simulink model "HDVSim_Dual_Fuel_Hybrid_Truck"  (R2018b)
settings: Solver=ode3  StartTime=0.0  StopTime=inf  FixedStep=sample_time  MaxStep=0.1  RelTol=1e-3  EnableMultiTasking=on
model workspace (MAT data in the model file):
  Bat : struct (value not decoded)
  Electric_Truck = 0
  Fueltype = 11
  Hybrid_Truck = 1
  IZ12 = 3600
  SOC_T_EM_completely_available = 0.089152566
  SOC_addition = 0.262901104
  SOC_target = 0
  Sailing_without_drag_torque = 1
  MCOS : class17 (value not decoded)
  TCO_Trailer = 1
  T_distance_LPS_down = 500
  T_distance_LPS_up = 434.9496342
  VSim : struct (value not decoded)
  Vehicle = 'LNGDieselHybrid'
  WPT : struct (value not decoded)
  MCOS : class17 (value not decoded)
  addition_for_critical_slope = 0.030662181
  ambient : struct (value not decoded)
  auxiliary_consumers : struct (value not decoded)
  critical_altitude_difference = 39.0505026
  cycle : struct (value not decoded)
  dcycle = 5
  distance_1_PPC = 130
  distance_2_PPC = 290
  distance_PPC_altitude_difference = 4273.353363
  driver : struct (value not decoded)
  em : struct (value not decoded)
  engine : struct (value not decoded)
  final_drive : struct (value not decoded)
  ifElectric = 0
  ifOptimized = 1
  look_ahead_PPC = 920
  max_distance = 3000
  name = 'HDVSim_Dual_Fuel_Hybrid_Truck'
  preditiveCruiseControl = 1
  sample_time = 0.1
  tank : struct (value not decoded)
  tires : struct (value not decoded)
  transmission : struct (value not decoded)
  v_PPC_delta = 2.77123754361
  v_max_electrical_drive_only = 9.22694367778
  vehicle : struct (value not decoded)
  MCOS : class17 (value not decoded)
  MCOS : class17 (value not decoded)
  x = [17.07936487 6 0 0 2.860669464 1810.391452 1020.247354 1265.144022 9.976455157 83 4 20 ... (27 elements, 1x27)]
values from neighbouring files (symbols this model uses):
  transmission = Transmission_gearing(1, 1, false, false, final_drive.ratio)    [Parameterizing.m]
symbols that are objects in the model workspace (value not decoded): ambient, auxiliary_consumers, Bat, cycle, driver, em, engine, final_drive, tires, vehicle
undefined symbols (not defined in the file or in its folder): Hybrid_LKW, Ion, Lithium
libraries: simulink x22, powerlib x2, electricdrivelib x1
(part 2 of 3)

== system HDVSim_Dual_Fuel_Hybrid_Truck/Active cruise control/Estimate acceleration ==
  v_target [m/s] : Inport
  Slope_0 : Inport  Port=2
  Slope_50 : Inport  Port=3
  Slope_100 : Inport  Port=4
  Slope_150 : Inport  Port=5
  Slope_200 : Inport  Port=6
  "Steigung_250 " : Inport  Port=7
  Slope_300 : Inport  Port=8
  Slope_350 : Inport  Port=9
  Slope_400 : Inport  Port=10
  Slope_450 : Inport  Port=11
  Add4 : Sum
  Constant4 : Constant  Value=vehicle.payload
  Constant9 : Constant  Value=vehicle.mass
  Demux : Demux  Outputs=10
  Divide1 : Product  Inputs=*/
  Driving resistance without acceleration : Subsystem
  Gain1 : Gain  Gain=-1
  Mux : Mux  Inputs=10
  Trigonometric Function2 : Trigonometry  Operator=atan
  Acceleration_0 : Outport
  Acceleration_50 : Outport  Port=2
  Acceleration_100 : Outport  Port=3
  Acceleration_150 : Outport  Port=4
  Acceleration_200 : Outport  Port=5
  Acceleration_250 : Outport  Port=6
  Acceleration_300 : Outport  Port=7
  Acceleration_350 : Outport  Port=8
  Acceleration_400 : Outport  Port=9
  Acceleration_450 : Outport  Port=10
  wires:
  v_target [m/s]/1 -> Driving resistance without acceleration/1(v [m/s])
  Trigonometric Function2/1 -> Driving resistance without acceleration/2(alpha [rad])
  Constant9/1 -> Add4/1
  Constant4/1 -> Add4/2
  Driving resistance without acceleration/1(F_x (resist) [N]) -> Gain1/1
  Add4/1 -> Divide1/2
  Gain1/1 -> Divide1/1
  Mux/1 -> Trigonometric Function2/1
  Divide1/1 -> Demux/1
  Demux/1 -> Acceleration_0/1
  Slope_0/1 -> Mux/1
  Slope_50/1 -> Mux/2
  Slope_100/1 -> Mux/3
  Slope_150/1 -> Mux/4
  Slope_200/1 -> Mux/5
  "Steigung_250 "/1 -> Mux/6
  Slope_300/1 -> Mux/7
  Slope_350/1 -> Mux/8
  Slope_400/1 -> Mux/9
  Slope_450/1 -> Mux/10
  Demux/2 -> Acceleration_50/1
  Demux/3 -> Acceleration_100/1
  Demux/4 -> Acceleration_150/1
  Demux/5 -> Acceleration_200/1
  Demux/6 -> Acceleration_250/1
  Demux/7 -> Acceleration_300/1
  Demux/8 -> Acceleration_350/1
  Demux/9 -> Acceleration_400/1
  Demux/10 -> Acceleration_450/1

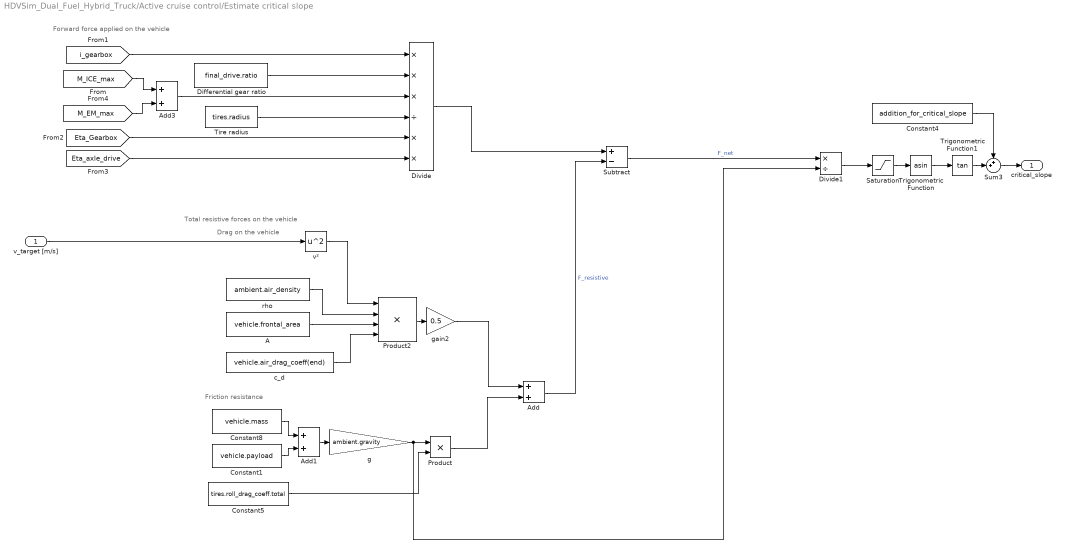
== system HDVSim_Dual_Fuel_Hybrid_Truck/Active cruise control/Estimate critical slope ==
  note: Total resistive forces on the vehicle
  note: Friction resistance
  note: Drag on the vehicle
  note: Forward force applied on the vehicle
  v_target [m/s] : Inport
  A : Constant  Value=vehicle.frontal_area
  Add : Sum
  Add1 : Sum
  Add3 : Sum
  Constant1 : Constant  Value=vehicle.payload
  Constant4 : Constant  Value=addition_for_critical_slope
  Constant5 : Constant  Value=tires.roll_drag_coeff.total
  Constant8 : Constant  Value=vehicle.mass
  Differential gear ratio : Constant  Value=final_drive.ratio
  Divide : Product  Inputs=***/**
  Divide1 : Product  Inputs=*/
  Product : Product
  Product2 : Product  Inputs=4  RndMeth=Zero
  Saturation : Saturate  UpperLimit=1  LowerLimit=-1
  Subtract : Sum  Inputs=+-
  Sum3 : Sum  Inputs=++|
  Tire radius : Constant  Value=tires.radius
  Trigonometric Function : Trigonometry  Operator=asin
  Trigonometric Function1 : Trigonometry  Operator=tan
  c_d : Constant  Value=vehicle.air_drag_coeff(end)
  g : Gain  Gain=ambient.gravity
  gain2 : Gain  Gain=0.5
  rho : Constant  Value=ambient.air_density
  v² : Math  Operator=square  SaturateOnIntegerOverflow=on
  critical_slope : Outport
  wires:
  Add3/1 -> Divide/3
  [i_gearbox] -> Divide/1
  Differential gear ratio/1 -> Divide/2
  Tire radius/1 -> Divide/4
  Divide/1 -> Subtract/1
  Subtract/1 -> Divide1/1  "F_net"
  v²/1 -> Product2/1
  rho/1 -> Product2/2
  A/1 -> Product2/3
  c_d/1 -> Product2/4
  Product2/1 -> gain2/1
  Constant8/1 -> Add1/1
  Constant1/1 -> Add1/2
  Add1/1 -> g/1
  Constant5/1 -> Product/2
  Trigonometric Function/1 -> Trigonometric Function1/1
  Divide1/1 -> Saturation/1
  Sum3/1 -> critical_slope/1
  Constant4/1 -> Sum3/1
  Trigonometric Function1/1 -> Sum3/2
  v_target [m/s]/1 -> v²/1
  [Eta_Gearbox] -> Divide/5
  [Eta_axle_drive] -> Divide/6
  [M_ICE_max] -> Add3/1
  [M_EM_max] -> Add3/2
  gain2/1 -> Add/1
  Product/1 -> Add/2
  Add/1 -> Subtract/2  "F_resistive"
  g/1 -> Product/1, Divide1/2
  Saturation/1 -> Trigonometric Function/1

== system HDVSim_Dual_Fuel_Hybrid_Truck/Active cruise control_old/Braking from upper speed limit ==
  v_soll [m/s] : Inport
  Add3 : Sum  Inputs=+-
  Constant1 : Constant  Value=90/3.6
  Constant10 : Constant  Value=preditiveCruiseControl
  Constant6 : Constant  Value=v_PPC_delta
  Constant7 : Constant  Value=0
  Constant8 : Constant  Value=0
  Saturation Dynamic : simulink/Discontinuities/Saturation Dynamic  OutMin=[]  OutMax=[]  OutDataTypeStr=Inherit: Same as second input  OutDataType=fixdt(1, 16)  OutScaling=2^-10  DoSatur=off
  Switch3 : Switch  Criteria=u2 > Threshold
  Out1 : Outport
  wires:
  Switch3/1 -> Out1/1
  Constant6/1 -> Saturation Dynamic/2
  Constant1/1 -> Add3/1
  Constant7/1 -> Switch3/3
  Add3/1 -> Saturation Dynamic/1
  Constant8/1 -> Saturation Dynamic/3
  Constant10/1 -> Switch3/2
  v_soll [m/s]/1 -> Add3/2
  Saturation Dynamic/1 -> Switch3/1

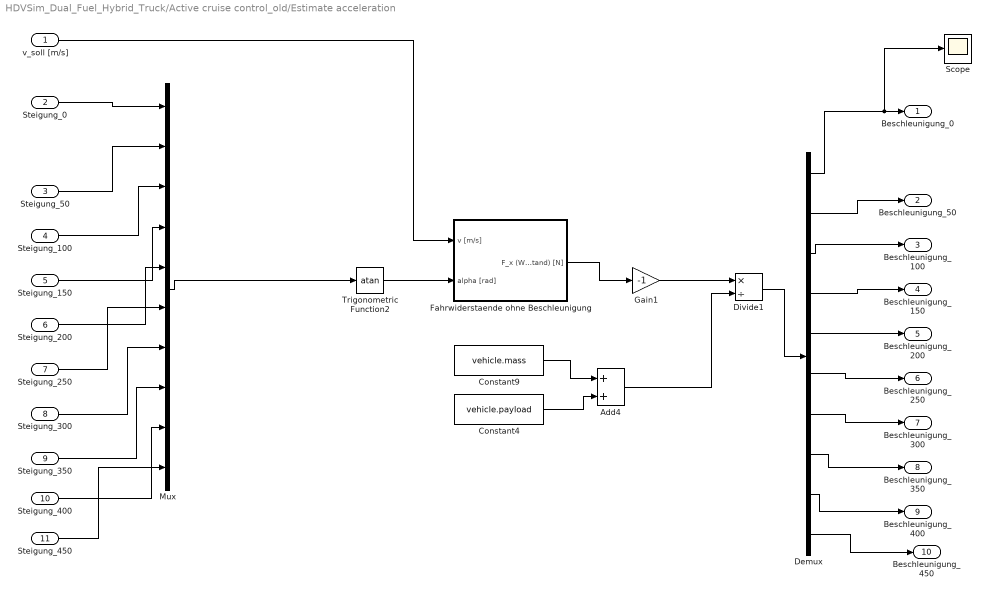
== system HDVSim_Dual_Fuel_Hybrid_Truck/Active cruise control_old/Estimate acceleration ==
  v_soll [m/s] : Inport
  Steigung_0 : Inport  Port=2
  Steigung_50 : Inport  Port=3
  Steigung_100 : Inport  Port=4
  Steigung_150 : Inport  Port=5
  Steigung_200 : Inport  Port=6
  "Steigung_250 " : Inport  Port=7
  Steigung_300 : Inport  Port=8
  Steigung_350 : Inport  Port=9
  Steigung_400 : Inport  Port=10
  Steigung_450 : Inport  Port=11
  Add4 : Sum
  Constant4 : Constant  Value=vehicle.payload
  Constant9 : Constant  Value=vehicle.mass
  Demux : Demux  Outputs=10
  Divide1 : Product  Inputs=*/
  Fahrwiderstaende ohne Beschleunigung : Subsystem
  Gain1 : Gain  Gain=-1
  Mux : Mux  Inputs=10
  Scope : Scope
  Trigonometric Function2 : Trigonometry  Operator=atan
  Beschleunigung_0 : Outport
  Beschleunigung_50 : Outport  Port=2
  Beschleunigung_100 : Outport  Port=3
  Beschleunigung_150 : Outport  Port=4
  Beschleunigung_200 : Outport  Port=5
  Beschleunigung_250 : Outport  Port=6
  Beschleunigung_300 : Outport  Port=7
  Beschleunigung_350 : Outport  Port=8
  Beschleunigung_400 : Outport  Port=9
  Beschleunigung_450 : Outport  Port=10
  wires:
  v_soll [m/s]/1 -> Fahrwiderstaende ohne Beschleunigung/1(v [m/s])
  Trigonometric Function2/1 -> Fahrwiderstaende ohne Beschleunigung/2(alpha [rad])
  Constant9/1 -> Add4/1
  Constant4/1 -> Add4/2
  Fahrwiderstaende ohne Beschleunigung/1(F_x (Widerstand) [N]) -> Gain1/1
  Add4/1 -> Divide1/2
  Gain1/1 -> Divide1/1
  Mux/1 -> Trigonometric Function2/1
  Divide1/1 -> Demux/1
  Demux/1 -> Scope/1, Beschleunigung_0/1
  Steigung_0/1 -> Mux/1
  Steigung_50/1 -> Mux/2
  Steigung_100/1 -> Mux/3
  Steigung_150/1 -> Mux/4
  Steigung_200/1 -> Mux/5
  "Steigung_250 "/1 -> Mux/6
  Steigung_300/1 -> Mux/7
  Steigung_350/1 -> Mux/8
  Steigung_400/1 -> Mux/9
  Steigung_450/1 -> Mux/10
  Demux/2 -> Beschleunigung_50/1
  Demux/3 -> Beschleunigung_100/1
  Demux/4 -> Beschleunigung_150/1
  Demux/5 -> Beschleunigung_200/1
  Demux/6 -> Beschleunigung_250/1
  Demux/7 -> Beschleunigung_300/1
  Demux/8 -> Beschleunigung_350/1
  Demux/9 -> Beschleunigung_400/1
  Demux/10 -> Beschleunigung_450/1

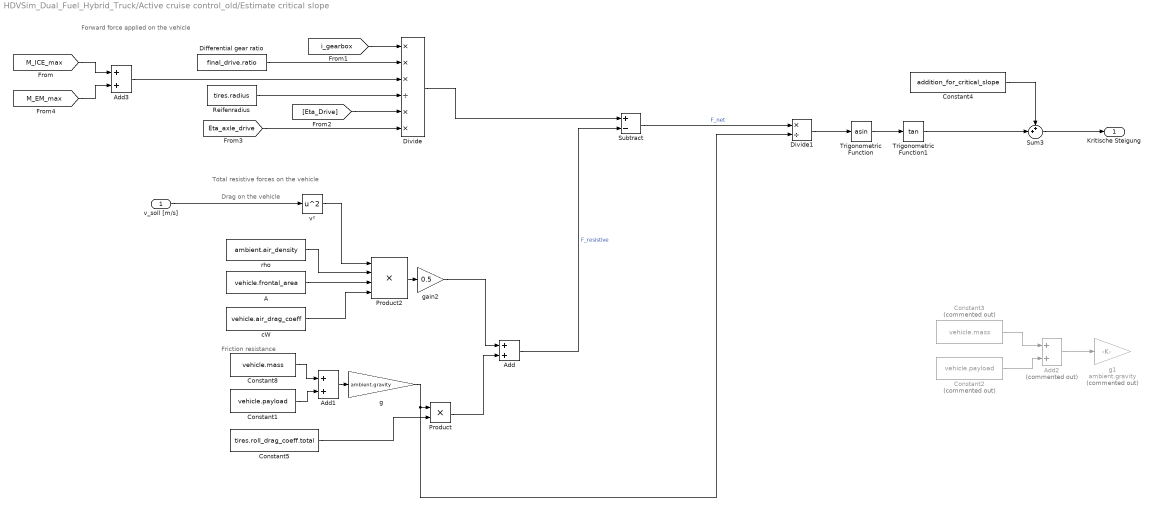
== system HDVSim_Dual_Fuel_Hybrid_Truck/Active cruise control_old/Estimate critical slope ==
  note: Forward force applied on the vehicle
  note: Drag on the vehicle
  note: Friction resistance
  note: Total resistive forces on the vehicle
  v_soll [m/s] : Inport
  A : Constant  Value=vehicle.frontal_area
  Add : Sum
  Add1 : Sum
  Add2 : Sum  Commented=on
  Add3 : Sum
  Constant1 : Constant  Value=vehicle.payload
  Constant2 : Constant  Commented=on  Value=vehicle.payload
  Constant3 : Constant  Commented=on  Value=vehicle.mass
  Constant4 : Constant  Value=addition_for_critical_slope
  Constant5 : Constant  Value=tires.roll_drag_coeff.total
  Constant8 : Constant  Value=vehicle.mass
  Differential gear ratio : Constant  Value=final_drive.ratio
  Divide : Product  Inputs=***/**
  Divide1 : Product  Inputs=*/
  Product : Product
  Product2 : Product  Inputs=4  RndMeth=Zero
  Reifenradius : Constant  Value=tires.radius
  Subtract : Sum  Inputs=+-
  Sum3 : Sum  Inputs=++|
  Trigonometric Function : Trigonometry  Operator=asin
  Trigonometric Function1 : Trigonometry  Operator=tan
  cW : Constant  Value=vehicle.air_drag_coeff
  g : Gain  Gain=ambient.gravity
  g1 : Gain  Commented=on  Gain=ambient.gravity
  gain2 : Gain  Gain=0.5
  rho : Constant  Value=ambient.air_density
  v² : Math  Operator=square  SaturateOnIntegerOverflow=on
  Kritische Steigung : Outport
  wires:
  Add3/1 -> Divide/3
  [i_gearbox] -> Divide/1
  Differential gear ratio/1 -> Divide/2
  Reifenradius/1 -> Divide/4
  Divide/1 -> Subtract/1
  v²/1 -> Product2/1
  rho/1 -> Product2/2
  A/1 -> Product2/3
  cW/1 -> Product2/4
  Product2/1 -> gain2/1
  Constant8/1 -> Add1/1
  Constant1/1 -> Add1/2
  Add1/1 -> g/1
  g/1 -> Divide1/2, Product/1
  Constant5/1 -> Product/2
  Constant3/1 -> Add2/1
  Constant2/1 -> Add2/2
  Add2/1 -> g1/1
  Trigonometric Function/1 -> Trigonometric Function1/1
  Divide1/1 -> Trigonometric Function/1
  Sum3/1 -> Kritische Steigung/1
  Constant4/1 -> Sum3/1
  Trigonometric Function1/1 -> Sum3/2
  v_soll [m/s]/1 -> v²/1
  [Eta_Drive] -> Divide/5
  [Eta_axle_drive] -> Divide/6
  [M_ICE_max] -> Add3/1
  [M_EM_max] -> Add3/2
  gain2/1 -> Add/1
  Product/1 -> Add/2
  Add/1 -> Subtract/2  "F_resistive"
  Subtract/1 -> Divide1/1  "F_net"

== system HDVSim_Dual_Fuel_Hybrid_Truck/Driver controls/PI controller brake ==
  delta_v : Inport
  Add : Sum
  "I - controller " : Gain  Gain=driver.controller_integral_gain
  "Integrator, reset for sign change of delta v" : Integrator  ExternalReset=either  ZeroCross=off
  "P - controller " : Gain  Gain=driver.controller_proportional_gain
  F_target [N] : Outport
  wires:
  "Integrator, reset for sign change of delta v"/1 -> Add/2  "I_part"
  "I - controller "/1 -> "Integrator, reset for sign change of delta v"/1
  Add/1 -> F_target [N]/1  "F_target"
  "P - controller "/1 -> Add/1  "P_part"
  delta_v/1 -> "I - controller "/1, "Integrator, reset for sign change of delta v"/2, "P - controller "/1

== system HDVSim_Dual_Fuel_Hybrid_Truck/Driver controls/PI controller throttle1 ==
  delta_v : Inport
  Add : Sum
  "I - controller " : Gain  Gain=driver.controller_integral_gain
  "Integrator, reset for sign change of delta v" : Integrator  ExternalReset=either  ZeroCross=off
  "P - controller " : Gain  Gain=driver.controller_proportional_gain
  F_target [N] : Outport
  wires:
  "Integrator, reset for sign change of delta v"/1 -> Add/2  "I_part"
  "I - controller "/1 -> "Integrator, reset for sign change of delta v"/1
  Add/1 -> F_target [N]/1  "F_target"
  "P - controller "/1 -> Add/1  "P_partl"
  delta_v/1 -> "Integrator, reset for sign change of delta v"/2, "I - controller "/1, "P - controller "/1

== system HDVSim_Dual_Fuel_Hybrid_Truck/Driver controls/ZKU ==
  In1 : Inport
  Switch1 : Switch  Threshold=1
  zero1 : Constant  Value=0
  Out1 : Outport
  wires:
  zero1/1 -> Switch1/1
  [ZKU] -> Switch1/2
  Switch1/1 -> Out1/1
  In1/1 -> Switch1/3

== system HDVSim_Dual_Fuel_Hybrid_Truck/Driver controls/ZKU1 ==
  In1 : Inport
  Switch1 : Switch  Threshold=1
  zero1 : Constant  Value=0
  Out1 : Outport
  wires:
  In1/1 -> Switch1/3
  Switch1/1 -> Out1/1
  [ZKU] -> Switch1/2
  zero1/1 -> Switch1/1

== system HDVSim_Dual_Fuel_Hybrid_Truck/Driving cycle/Holding time at the beginning ==
  In1 : Inport
  Clock2 : Clock
  Constant3 : Constant  Value=cycle.stop_start
  Constant4 : Constant  Value=0
  Subtract1 : Sum  Inputs=+-
  Switch1 : Switch
  Out1 : Outport
  wires:
  In1/1 -> Switch1/1
  Constant3/1 -> Subtract1/2
  Clock2/1 -> Subtract1/1
  Constant4/1 -> Switch1/3
  Subtract1/1 -> Switch1/2
  Switch1/1 -> Out1/1

== system HDVSim_Dual_Fuel_Hybrid_Truck/Driving cycle/Holding time at the end ==
  In1 : Inport
  Clock1 : Clock
  Constant : Constant
  Constant1 : Constant  Value=cycle.stop_end
  Constant2 : Constant
  Hit Crossing : HitCross  HitCrossingDirection=rising
  Integrator : Integrator  ExternalReset=rising
  Subtract : Sum  Inputs=+-
  Sum1 : Sum  Inputs=|++
  Switch : Switch  Criteria=u2 > Threshold  Threshold=cycle.stop_end
  Out1 : Outport
  wires:
  In1/1 -> Integrator/2
  Constant/1 -> Integrator/1
  Subtract/1 -> Hit Crossing/1
  Integrator/1 -> Switch/1
  Hit Crossing/1 -> Out1/1
  Clock1/1 -> Switch/2
  Constant1/1 -> Sum1/2, Subtract/2
  Sum1/1 -> Switch/3
  Switch/1 -> Subtract/1
  Constant2/1 -> Sum1/1

== system HDVSim_Dual_Fuel_Hybrid_Truck/Driving cycle/Significant speed deviation ==
  In1 : Inport
  Clock : Clock
  Compare To Constant : simulink/Logic and Bit Operations/Compare To Constant  relop=>=  const=30  OutDataTypeStr=boolean
  Compare To Constant1 : simulink/Logic and Bit Operations/Compare To Constant  relop=>=  const=1000  OutDataTypeStr=boolean
  Compare To Constant2 : simulink/Logic and Bit Operations/Compare To Constant  relop=<=  const=0.1  OutDataTypeStr=boolean
  Compare To Constant3 : simulink/Logic and Bit Operations/Compare To Constant  relop=>=  const=1000  OutDataTypeStr=boolean
  Constant : Constant
  Constant1 : Constant  Value=0
  Constant2 : Constant
  Constant3 : Constant  Value=0
  Display : Display
  Display1 : Display
  Display2 : Display
  Gain : Gain  Gain=3.6
  Gain1 : Gain  Gain=3.6
  Integrator1 : Integrator  ExternalReset=either
  Integrator2 : Integrator  ExternalReset=either
  Logical Operator : Logic  Operator=OR  AllPortsSameDT=off  OutDataTypeStr=boolean
  Sum : Sum  Inputs=|+-
  Switch : Switch  Criteria=u2 > Threshold
  Switch1 : Switch  Criteria=u2 > Threshold
  stop_time : Lookup_n-D  NumberOfTableDimensions=1  BreakpointsForDimension1=cycle.distance  Table=cycle.stop_time  InterpMethod=Flat  RndMeth=Simplest  InputSameDT=on
  Out1 : Outport
  wires:
  In1/1 -> stop_time/1
  stop_time/1 -> Sum/2
  [delta_v] -> Gain/1
  [v_actual_1] -> Gain1/1
  Gain/1 -> Compare To Constant/1
  Integrator2/1 -> Display/1, Compare To Constant1/1
  Compare To Constant1/1 -> Logical Operator/2
  Gain1/1 -> Compare To Constant2/1
  Integrator1/1 -> Sum/1
  Sum/1 -> Display1/1, Compare To Constant3/1
  Compare To Constant3/1 -> Logical Operator/1
  Logical Operator/1 -> Out1/1
  Switch1/1 -> Integrator2/1, Integrator2/2
  Switch/1 -> Integrator1/2, Integrator1/1
  Constant/1 -> Switch/1
  Compare To Constant2/1 -> Switch/2
  Constant1/1 -> Switch/3
  Constant2/1 -> Switch1/1
  Compare To Constant/1 -> Switch1/2
  Constant3/1 -> Switch1/3
  Clock/1 -> Display2/1

== system HDVSim_Dual_Fuel_Hybrid_Truck/ECU/Approach to stop ==
  stop_time [s] : Inport
  Clock : Clock
  Compare To Constant1 : simulink/Logic and Bit Operations/Compare To Constant  relop=<=  const=3  OutDataTypeStr=boolean
  Compare To Zero : simulink/Logic and Bit Operations/Compare To Zero  relop=<=  OutDataTypeStr=boolean
  Constant : Constant
  Constant1 : Constant  Value=3.1
  Constant2 : Constant
  Hit Crossing : HitCross  HitCrossingDirection=rising
  Integrator : Integrator  ExternalReset=rising  InitialCondition=0.001
  Integrator1 : Integrator  ExternalReset=rising
  Subtract : Sum  Inputs=+-
  Switch : Switch  Criteria=u2 > Threshold  Threshold=3
  Driver_M : Outport
  Driver_B : Outport  Port=2
  wires:
  Constant/1 -> Integrator/1
  stop_time [s]/1 -> Integrator/2, Subtract/2
  Integrator/1 -> Subtract/1
  Subtract/1 -> Compare To Zero/1, Hit Crossing/1
  Constant2/1 -> Integrator1/1
  Hit Crossing/1 -> Integrator1/2
  Clock/1 -> Switch/2
  Constant1/1 -> Switch/3
  Integrator1/1 -> Switch/1
  Switch/1 -> Compare To Constant1/1
  Compare To Constant1/1 -> Driver_M/1
  Compare To Zero/1 -> Driver_B/1

== system HDVSim_Dual_Fuel_Hybrid_Truck/ECU/Calculations for braking ==
  note: Breaking from motor's regenerative breaking
  note: Breaking from disk brakes
  M_EM_max [Nm] : Inport
  Driver_B : Inport  Port=2
  Gear : Inport  Port=3
  Differential efficiency : Constant  Value=final_drive.trq_eff
  Differential gear ratio : Constant  Value=final_drive.ratio
  Divide : Product  Inputs=*/
  Divide1 : Product  Inputs=**/*/
  Efficiencies : Lookup  InputValues=[1:length(transmission.ratios)]  Table=transmission.trq_eff  LookUpMeth=Use Input Nearest
  Gearing : Lookup  InputValues=[1:length(transmission.ratios)]  Table=transmission.ratios  LookUpMeth=Use Input Nearest
  Maximum breaking force [N] : Constant  Value=vehicle.F_brake_max
  Product : Product
  Time radius : Constant  Value=tires.radius
  F_brake_required [N] : Outport
  F_brake_elec_max [N] : Outport  Port=2
  wires:
  M_EM_max [Nm]/1 -> Divide1/1
  Divide/1 -> F_brake_elec_max [N]/1
  Divide1/1 -> Divide/1
  Time radius/1 -> Divide/2
  Driver_B/1 -> Product/1
  Maximum breaking force [N]/1 -> Product/2
  Product/1 -> F_brake_required [N]/1
  Gear/1 -> Efficiencies/1, Gearing/1
  Gearing/1 -> Divide1/2
  Efficiencies/1 -> Divide1/3
  Differential gear ratio/1 -> Divide1/4
  Differential efficiency/1 -> Divide1/5

== system HDVSim_Dual_Fuel_Hybrid_Truck/ECU/Calculations for throttle ==
  Driver_M : Inport
  SOC : Inport  Port=2
  n_ICE [rpm] : Inport  Port=3
  n_EM [rpm] : Inport  Port=4
  Constant : Constant  Value=SOC_T_EM_completely_available
  Constant1 : Constant  Value=0
  Divide : Product  Inputs=*/
  Divide1 : Product  Inputs=*/
  Drag torque : Lookup  InputValues=engine.drag_torque.speed  Table=engine.drag_torque.trq  LookUpMeth=Interpolation-Use End Values
  Electrical machine speed-torque characteristics : Lookup_n-D  NumberOfTableDimensions=1  BreakpointsForDimension1=em.speed  Table=em.trq  ExtrapMethod=Clip  RndMeth=Simplest  InputSameDT=on
  Gain : Gain  Gain=2*pi/60
  Memory : Memory
  Memory1 : Memory
  P_aux [W] : Constant  Value=auxiliary_consumers.power
  Product : Product
  Product1 : Product
  Saturation : Saturate  UpperLimit=inf  LowerLimit=0.001
  Saturation Dynamic : simulink/Discontinuities/Saturation Dynamic  OutMin=[]  OutMax=[]  OutDataTypeStr=Inherit: Same as second input  OutDataType=fixdt(1, 16)  OutScaling=2^-10  DoSatur=off
  Saturation1 : Saturate  UpperLimit=1000000  LowerLimit=0.0000001
  Sum1 : Sum  Inputs=|++
  Torque for be_min : Lookup_n-D  NumberOfTableDimensions=1  BreakpointsForDimension1=engine.bsfc.speed  Table=engine.bsfc.M_be_min  ExtrapMethod=Clip  RndMeth=Simplest  InputSameDT=on
  Volllastkurve : Lookup  InputValues=engine.full_load.speed  Table=engine.full_load.trq  LookUpMeth=Interpolation-Use End Values
  M_ICE_max [Nm] : Outport
  M_EM_max [Nm] : Outport  Port=2
  M_Required [Nm] : Outport  Port=3
  M_be_min [Nm] : Outport  Port=4
  M_Drag [Nm] : Outport  Port=5
  M_aux [Nm] : Outport  Port=6
  tag scope: M_EM_max=global, M_ICE_max=global
  wires:
  Volllastkurve/1 -> [M_ICE_max], Sum1/2, M_ICE_max [Nm]/1  "M_VM_max"
  Torque for be_min/1 -> M_be_min [Nm]/1
  Sum1/1 -> Product/2
  Product/1 -> M_Required [Nm]/1
  Drag torque/1 -> M_Drag [Nm]/1
  n_ICE [rpm]/1 -> Memory/1
  Gain/1 -> Divide/2
  P_aux [W]/1 -> Divide/1
  Divide/1 -> M_aux [Nm]/1
  Electrical machine speed-torque characteristics/1 -> [M_EM_max], Saturation Dynamic/1, M_EM_max [Nm]/1, Divide1/1
  Product1/1 -> Saturation Dynamic/2
  Saturation/1 -> Gain/1
  n_EM [rpm]/1 -> Memory1/1
  Memory/1 -> Saturation/1, Volllastkurve/1, Torque for be_min/1, Drag torque/1
  Memory1/1 -> Electrical machine speed-torque characteristics/1
  Constant/1 -> Divide1/2
  Saturation Dynamic/1 -> Sum1/1
  Constant1/1 -> Saturation Dynamic/3
  SOC/1 -> Product1/2
  Driver_M/1 -> Product/1
  Divide1/1 -> Saturation1/1
  Saturation1/1 -> Product1/1

== system HDVSim_Dual_Fuel_Hybrid_Truck/Electric motor/Machine current demand ==
  note: Electric power calculation
  "n_EM " : Inport
  M_EM_target [Nm] : Inport  Port=2
  Eff_EM : Inport  Port=3
  U_Bat [V] : Inport  Port=4
  Divide : Product  Inputs=*/*
  Divide1 : Product  Inputs=*/
  Gain : Gain  Gain=2*pi/60
  Saturation1 : Saturate  UpperLimit=inf  LowerLimit=1
  I_target [A] : Outport
  wires:
  Divide/1 -> Divide1/1
  Divide1/1 -> I_target [A]/1
  Gain/1 -> Divide/3
  M_EM_target [Nm]/1 -> Divide/1
  "n_EM "/1 -> Saturation1/1
  U_Bat [V]/1 -> Divide1/2
  Eff_EM/1 -> Divide/2
  Saturation1/1 -> Gain/1

== system HDVSim_Dual_Fuel_Hybrid_Truck/Electric motor/Machine torque demand ==
  n_EM [rpm] : Inport
  I_current [A] : Inport  Port=2
  Eff_EM : Inport  Port=3
  U_Bat [V] : Inport  Port=4
  Divide : Product  Inputs=*/*
  Gain : Gain  Gain=2*pi/60
  Product : Product
  Saturation1 : Saturate  UpperLimit=inf  LowerLimit=1
  M_EM [Nm] : Outport
  wires:
  U_Bat [V]/1 -> Product/1
  n_EM [rpm]/1 -> Saturation1/1
  Product/1 -> Divide/1
  Gain/1 -> Divide/2
  Divide/1 -> M_EM [Nm]/1
  I_current [A]/1 -> Product/2
  Eff_EM/1 -> Divide/3
  Saturation1/1 -> Gain/1

== system HDVSim_Dual_Fuel_Hybrid_Truck/ICE engine/Additional consumptions ==
  M_ICE_bfor_aux [Nm] : Inport
  n_clutch_en [rpm] : Inport  Port=2
  "1/min -> 1/s" : Gain  Gain=1/60
  2*pi : Constant  Value=2*pi
  M_ICE_bfor_aux - M_aux [Nm] : Sum  Inputs=+-
  P_aux [W] : Constant  Value=auxiliary_consumers.power
  Product1 : Product  Inputs=*//  RndMeth=Zero
  M_ICE_aftr_aux [Nm] : Outport
  wires:
  n_clutch_en [rpm]/1 -> "1/min -> 1/s"/1
  "1/min -> 1/s"/1 -> Product1/3
  2*pi/1 -> Product1/2
  P_aux [W]/1 -> Product1/1
  Product1/1 -> M_ICE_bfor_aux - M_aux [Nm]/2  "M_NV"
  M_ICE_bfor_aux [Nm]/1 -> M_ICE_bfor_aux - M_aux [Nm]/1
  M_ICE_bfor_aux - M_aux [Nm]/1 -> M_ICE_aftr_aux [Nm]/1

== system HDVSim_Dual_Fuel_Hybrid_Truck/ICE engine/Consumption ==
  note: Amounts of each fuel
  note: Fuel mass flow
  note: Total fuel amount calculation
  M [Nm] : Inport
  n [rpm] : Inport  Port=2
  Compare To Constant : simulink/Logic and Bit Operations/Compare To Constant  relop=>=  const=0.3  OutDataTypeStr=uint8  ZeroCross=off
  Compare To Zero : simulink/Logic and Bit Operations/Compare To Zero  relop=<=  OutDataTypeStr=uint8  ZeroCross=off
  Constant : Constant  Value=0
  Divide : Product  Inputs=/*
  Engine torque-speed table : Lookup_n-D  BreakpointsForDimension1=engine.bsfc.trq  BreakpointsForDimension2=engine.bsfc.speed  BeginIndexSearchUsingPreviousIndexResult=on  Table=engine.bsfc.be  TableMin=[0]  TableMax=[1]  InterpMethod=Cubic spline  ExtrapMethod=Clip  InternalRulePriority=Speed  RndMeth=Nearest
  Fuel economy [Liter/100km] : Subsystem
  Gain : Gain  Gain=0.94
  Gain1 : Gain  Gain=0.06
  Gain2 : Gain  Gain=1/engine.fuel.density_diesel
  Idle consumption : Constant  Value=engine.idle_fuel_consumption
  Integrator : Integrator
  MinMax : MinMax  Function=max  Inputs=2  ZeroCross=off
  Product5 : Product  RndMeth=Zero
  Saturation1 : Saturate  UpperLimit=engine.M_max  LowerLimit=0  ZeroCross=off
  Switch : Switch  Threshold=1  ZeroCross=off
  g/h->l/h : Gain  Gain=1/engine.fuel.heat_of_combustion
  kg/h->kg/s : Gain  Gain=1/3600
  m->km : Gain  Gain=1/1000
  "n->omega, min->s" : Gain  Gain=pi/30000
  tag scope: Consumption_absolut_LNG_kg=global, Consumption_absolut_diesel_l=global, Consumption_diesel_l_per_100km=global, Consumption_gas_kg_per_100km=global
  wires:
  [s_actual_1] -> m->km/1
  Fuel economy [Liter/100km]/1(Diesel consumption l/100km) -> [Consumption_diesel_l_per_100km]  "Fuel economy [l/100km]"
  m->km/1 -> Compare To Constant/1, Fuel economy [Liter/100km]/3(s [km])
  Compare To Constant/1 -> Fuel economy [Liter/100km]/Enable
  n [rpm]/1 -> Engine torque-speed table/2, Product5/2
  Product5/1 -> "n->omega, min->s"/1
  Divide/1 -> g/h->l/h/1  "P_Kraftstoff [kW]"
  Engine torque-speed table/1 -> Divide/1  "eta"
  "n->omega, min->s"/1 -> Divide/2  "P_mot [kW]"
  g/h->l/h/1 -> MinMax/1  "m. [kg/s]"
  Switch/1 -> Integrator/1  "m. [kg/s]"
  Integrator/1 -> Gain/1, Gain1/1  "m [kg]"
  Idle consumption/1 -> kg/h->kg/s/1
  M [Nm]/1 -> Compare To Zero/1, Saturation1/1
  MinMax/1 -> Switch/3
  Constant/1 -> Switch/1
  Saturation1/1 -> Engine torque-speed table/1, Product5/1
  Compare To Zero/1 -> Switch/2
  kg/h->kg/s/1 -> MinMax/2
  Gain/1 -> Fuel economy [Liter/100km]/2(Gas consumption [kg]), [Consumption_absolut_LNG_kg]  "m_gas [kg]"
  Gain1/1 -> Gain2/1  "m_Diesel [kg]"
  Gain2/1 -> Fuel economy [Liter/100km]/1(abs Diesel consumption [l]), [Consumption_absolut_diesel_l]  "Volume_diesel [l]"
  Fuel economy [Liter/100km]/2(Gas economy [kg/100km]) -> [Consumption_gas_kg_per_100km]

== system HDVSim_Dual_Fuel_Hybrid_Truck/ICE engine/maximum engine torque due to tire slip ==
  note: Wheel torque
  note: Wheel torque after losses & multiplications
  note: Overall transmission efficiency
  note: Overall transmission gear ratio
  Constant1 : Constant  Value=vehicle.Fx_max
  Differential efficiency : Constant  Value=final_drive.trq_eff
  Differential ratio : Constant  Value=final_drive.ratio
  Efficiencies : Lookup  InputValues=[1:length(transmission.ratios)]  Table=transmission.trq_eff  LookUpMeth=Use Input Nearest
  Gearing : Lookup  InputValues=[1:length(transmission.ratios)]  Table=transmission.ratios  LookUpMeth=Use Input Nearest
  Product : Product  Inputs=*//  RndMeth=Zero
  Product1 : Product  RndMeth=Zero
  Product2 : Product  Inputs=*//  RndMeth=Zero
  Tire radius : Constant  Value=tires.radius
  M_mot_max_traction [Nm] : Outport
  wires:
  Tire radius/1 -> Product1/2
  Constant1/1 -> Product1/1
  [gear] -> Efficiencies/1, Gearing/1
  Product1/1 -> Product/1  "M_rad_max_traction"
  Efficiencies/1 -> Product/2
  Gearing/1 -> Product/3
  Product/1 -> Product2/1
  Differential efficiency/1 -> Product2/2
  Differential ratio/1 -> Product2/3
  Product2/1 -> M_mot_max_traction [Nm]/1

== system HDVSim_Dual_Fuel_Hybrid_Truck/Power electronics & battery/Conversion of SOC ==
  SOC_absolut : Inport
  Constant : Constant  Value=0.5-Bat.Useable_range/2
  Constant1 : Constant  Value=0.5+Bat.Useable_range/2
  Divide : Product  Inputs=*/
  Saturation : Saturate  UpperLimit=1  LowerLimit=0
  Sum : Sum  Inputs=+-
  Sum1 : Sum  Inputs=-+
  SOC_relative : Outport
  wires:
  SOC_absolut/1 -> Sum/1
  Constant/1 -> Sum1/1, Sum/2
  Sum/1 -> Divide/1
  Constant1/1 -> Sum1/2
  Sum1/1 -> Divide/2
  Divide/1 -> Saturation/1
  Saturation/1 -> SOC_relative/1

== system HDVSim_Dual_Fuel_Hybrid_Truck/Power electronics & battery/Power electronics ==
  I_PE_current [A] : Inport
  1/Eta_LE : Gain  Gain=1/Bat.Efficiency_power_electronics
  Eta_LE : Gain  Gain=Bat.Efficiency_power_electronics
  Switch : Switch  Criteria=u2 > Threshold
  I_BAT_current [A] : Outport
  wires:
  Eta_LE/1 -> Switch/1
  1/Eta_LE/1 -> Switch/3
  I_PE_current [A]/1 -> 1/Eta_LE/1, Eta_LE/1, Switch/2
  Switch/1 -> I_BAT_current [A]/1

== system HDVSim_Dual_Fuel_Hybrid_Truck/Power electronics & battery/To prevent division by zero ==
  In1 : Inport
  In2 : Inport  Port=2
  In3 : Inport  Port=3
  Enable : EnablePort
  Abs : Abs
  Divide1 : Product  Inputs=*/
  Product1 : Product
  Out1 : Outport
  wires:
  In2/1 -> Product1/1
  In1/1 -> Product1/2
  In3/1 -> Divide1/1
  Product1/1 -> Divide1/2
  Divide1/1 -> Abs/1
  Abs/1 -> Out1/1  "Losses (%)"

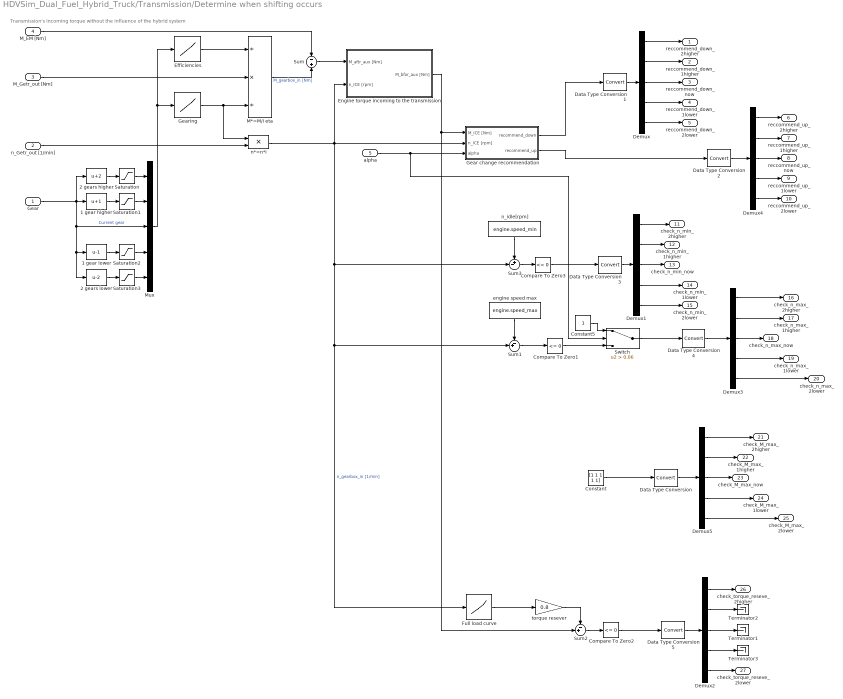
== system HDVSim_Dual_Fuel_Hybrid_Truck/Transmission/Determine when shifting occurs ==
  note: Transmission's incoming torque without the influence of the hybrid system
  Gear : Inport
  n_Getr_out [1/min] : Inport  Port=2
  M_Getr_out [Nm] : Inport  Port=3
  M_EM [Nm] : Inport  Port=4
  alpha : Inport  Port=5
  1 gear higher : Bias  Bias=1
  1 gear lower : Bias  Bias=-1
  2 gears higher : Bias  Bias=2
  2 gears lower : Bias  Bias=-2
  Compare To Zero1 : simulink/Logic and Bit Operations/Compare To Zero  relop=<=  OutDataTypeStr=boolean
  Compare To Zero2 : simulink/Logic and Bit Operations/Compare To Zero  relop=<=  OutDataTypeStr=boolean
  Compare To Zero3 : simulink/Logic and Bit Operations/Compare To Zero  relop=<=  OutDataTypeStr=boolean
  Constant : Constant  Value=[1 1 1 1 1]
  Constant5 : Constant
  Data Type Conversion{,1..5} (6 alike) : DataTypeConversion
  Demux{,1..5} (6 alike) : Demux  Outputs=5
  Efficiencies : Lookup  InputValues=[1:length(transmission.ratios)]  Table=transmission.trq_eff  LookUpMeth=Use Input Nearest
  Engine torque incoming to the transmission : Subsystem
  Full load curve : Lookup  InputValues=engine.full_load.speed  Table=engine.full_load.trq  LookUpMeth=Interpolation-Use End Values
  Gear change recommendation : Subsystem
  Gearing : Lookup  InputValues=[1:length(transmission.ratios)]  Table=transmission.ratios  LookUpMeth=Use Input Nearest
  M*=M/i eta : Product  Inputs=/*/
  Mux : Mux  Inputs=5
  Saturation{,1..3} (4 alike) : Saturate  UpperLimit=length(transmission.ratios)  LowerLimit=0
  Sum : Sum  Inputs=-+
  Sum1 : Sum  Inputs=-+|
  Sum2 : Sum  Inputs=-+|
  Sum3 : Sum  Inputs=+-|
  Switch : Switch  Criteria=u2 > Threshold  Threshold=0.06
  Terminator1 : Terminator
  Terminator2 : Terminator
  Terminator3 : Terminator
  engine speed max : Constant  Value=engine.speed_max
  n*=n*i : Product  Inputs=**
  n_idle[rpm] : Constant  Value=engine.speed_min
  torque resever : Gain  Gain=0.8
  reccommend_down_2higher : Outport
  reccommend_down_1higher : Outport  Port=2
  reccommend_down_now : Outport  Port=3
  reccommend_down_1lower : Outport  Port=4
  reccommend_down_2lower : Outport  Port=5
  reccommend_up_2higher : Outport  Port=6
  reccommend_up_1higher : Outport  Port=7
  reccommend_up_now : Outport  Port=8
  reccommend_up_1lower : Outport  Port=9
  reccommend_up_2lower : Outport  Port=10
  check_n_min_2higher : Outport  Port=11
  check_n_min_1higher : Outport  Port=12
  check_n_min_now : Outport  Port=13
  check_n_min_1lower : Outport  Port=14
  check_n_min_2lower : Outport  Port=15
  check_n_max_2higher : Outport  Port=16
  check_n_max_1higher : Outport  Port=17
  check_n_max_now : Outport  Port=18
  check_n_max_1lower : Outport  Port=19
  check_n_max_2lower : Outport  Port=20
  check_M_max_2higher : Outport  Port=21
  check_M_max_1higher : Outport  Port=22
  check_M_max_now : Outport  Port=23
  check_M_max_1lower : Outport  Port=24
  check_M_max_2lower : Outport  Port=25
  check_torque_reseve_2higher : Outport  Port=26
  check_torque_reseve_2lower : Outport  Port=27
  wires:
  Gear/1 -> 1 gear higher/1, Mux/3, 1 gear lower/1, 2 gears lower/1, 2 gears higher/1  "Current gear"
  Engine torque incoming to the transmission/1(M_bfor_aux [Nm]) -> Sum2/2, Gear change recommendation/1(M_ICE [Nm])
  n*=n*i/1 -> Engine torque incoming to the transmission/2(n_ICE [rpm]), Gear change recommendation/2(n_ICE [rpm]), Full load curve/1, Sum1/2, Sum3/2  "n_gearbox_in [1/min]"
  n_Getr_out [1/min]/1 -> n*=n*i/2
  Efficiencies/1 -> M*=M/i eta/1
  M_Getr_out [Nm]/1 -> M*=M/i eta/2
  2 gears higher/1 -> Saturation/1
  1 gear higher/1 -> Saturation1/1
  Mux/1 -> Efficiencies/1, Gearing/1
  Demux/1 -> reccommend_down_2higher/1
  Demux/2 -> reccommend_down_1higher/1
  Demux/3 -> reccommend_down_now/1
  Demux2/1 -> check_torque_reseve_2higher/1
  Demux2/2 -> Terminator2/1
  Demux2/3 -> Terminator1/1
  Demux1/1 -> check_n_min_2higher/1
  Demux1/2 -> check_n_min_1higher/1
  Demux1/3 -> check_n_min_now/1
  Gearing/1 -> M*=M/i eta/3, n*=n*i/1
  Saturation/1 -> Mux/1
  Saturation1/1 -> Mux/2
  1 gear lower/1 -> Saturation2/1
  Saturation2/1 -> Mux/4
  2 gears lower/1 -> Saturation3/1
  Saturation3/1 -> Mux/5
  Demux2/4 -> Terminator3/1
  Demux2/5 -> check_torque_reseve_2lower/1
  Demux/5 -> reccommend_down_2lower/1
  Demux/4 -> reccommend_down_1lower/1
  Demux1/4 -> check_n_min_1lower/1
  Demux1/5 -> check_n_min_2lower/1
  Demux4/1 -> reccommend_up_2higher/1
  Demux4/2 -> reccommend_up_1higher/1
  Demux4/3 -> reccommend_up_now/1
  Demux4/5 -> reccommend_up_2lower/1
  Demux4/4 -> reccommend_up_1lower/1
  Gear change recommendation/1(recommend_down) -> Data Type Conversion1/1
  Full load curve/1 -> torque resever/1
  torque resever/1 -> Sum2/1
  Sum2/1 -> Compare To Zero2/1
  Sum3/1 -> Compare To Zero3/1
  n_idle[rpm]/1 -> Sum3/1
  Compare To Zero3/1 -> Data Type Conversion3/1
  Gear change recommendation/2(recommend_up) -> Data Type Conversion2/1
  Demux3/1 -> check_n_max_2higher/1
  Demux3/2 -> check_n_max_1higher/1
  Demux3/3 -> check_n_max_now/1
  Demux3/4 -> check_n_max_1lower/1
  Demux3/5 -> check_n_max_2lower/1
  Sum1/1 -> Compare To Zero1/1
  engine speed max/1 -> Sum1/1
  Demux5/1 -> check_M_max_2higher/1
  Demux5/2 -> check_M_max_1higher/1
  Demux5/3 -> check_M_max_now/1
  Demux5/4 -> check_M_max_1lower/1
  Demux5/5 -> check_M_max_2lower/1
  Data Type Conversion1/1 -> Demux/1
  Data Type Conversion2/1 -> Demux4/1
  Data Type Conversion3/1 -> Demux1/1
  Data Type Conversion4/1 -> Demux3/1
  Data Type Conversion5/1 -> Demux2/1
  Constant/1 -> Data Type Conversion/1
  Sum/1 -> Engine torque incoming to the transmission/1(M_aftr_aux [Nm])
  M*=M/i eta/1 -> Sum/2  "M_gearbox_in [Nm]"
  M_EM [Nm]/1 -> Sum/1
  alpha/1 -> Switch/2, Gear change recommendation/3(alpha)
  Constant5/1 -> Switch/1
  Compare To Zero1/1 -> Switch/3
  Data Type Conversion/1 -> Demux5/1
  Switch/1 -> Data Type Conversion4/1
  Compare To Zero2/1 -> Data Type Conversion5/1

== system HDVSim_Dual_Fuel_Hybrid_Truck/Transmission/Torque flow through the transmission ==
  note: Rotational speed before and after the transmission
  note: Outgoing torque from the transmission
  M_gearbox_in [Nm] : Inport
  n_gearbox_out [1/min] : Inport  Port=2
  Gear : Inport  Port=3
  Divide : Product  Inputs=/
  Efficiencies : Lookup  InputValues=[1:length(transmission.ratios)]  Table=transmission.trq_eff  LookUpMeth=Use Input Nearest
  Gearing : Lookup  InputValues=[1:length(transmission.ratios)]  Table=transmission.ratios  LookUpMeth=Use Input Nearest
  M_Mot >= 0? : Switch  ZeroCross=off
  Product : Product  Inputs=***  RndMeth=Zero
  Rotating mass : Lookup  InputValues=[1:length(transmission.ratios)]  Table=transmission.lamda  LookUpMeth=Use Input Nearest
  n*=n*i : Product  Inputs=**
  n_gearbox_in [1/min] : Outport
  M_gearbox_out [Nm] : Outport  Port=2
  i_gearbox : Outport  Port=3
  tag scope: Eta_Gearbox=global, lamda=global
  wires:
  Gearing/1 -> n*=n*i/1, i_gearbox/1, Product/3  "Gear ratios"
  n*=n*i/1 -> n_gearbox_in [1/min]/1
  Rotating mass/1 -> [lamda]  "lambda"
  n_gearbox_out [1/min]/1 -> n*=n*i/2
  Gear/1 -> Gearing/1, Rotating mass/1, Efficiencies/1
  M_gearbox_in [Nm]/1 -> M_Mot >= 0?/2, Product/2
  Product/1 -> M_gearbox_out [Nm]/1
  Efficiencies/1 -> Divide/1, M_Mot >= 0?/1  "Eta_Gear"
  Divide/1 -> M_Mot >= 0?/3
  M_Mot >= 0?/1 -> Product/1, [Eta_Gearbox]

== system HDVSim_Dual_Fuel_Hybrid_Truck/Transmission/ZKU ==
  Gear : Inport
  Compare : simulink/Logic and Bit Operations/Compare To Zero  relop=>=  OutDataTypeStr=uint8  ZeroCross=off
  Constant : Constant  Value=-1
  Constant1 : Constant  Value=0
  Constant2 : Constant  Value=0
  Data Type Conversion : DataTypeConversion
  Derivative : Derivative
  Integrator : Integrator  ExternalReset=either  InitialCondition=transmission.shift_time
  Manual Switch : ManualSwitch
  Memory : Memory
  Switch : Switch  Threshold=1
  tag scope: ZKU=global
  wires:
  Constant/1 -> Integrator/1
  Derivative/1 -> Integrator/2
  Integrator/1 -> Compare/1
  Compare/1 -> Data Type Conversion/1
  Data Type Conversion/1 -> Switch/3
  Constant1/1 -> Manual Switch/2
  Gear/1 -> Manual Switch/1
  Manual Switch/1 -> Derivative/1
  [E_DRIVING] -> Switch/2
  Constant2/1 -> Switch/1
  Switch/1 -> Memory/1
  Memory/1 -> [ZKU]

== system HDVSim_Dual_Fuel_Hybrid_Truck/Vehicle/Driving resistances without acceleration ==
  alpha [rad] : Inport
  v [m/s] : Inport  Port=2
  Add : Sum  Inputs=+++
  Drag : Subsystem
  Gradient resistance : Subsystem
  Rolling resistance : Subsystem
  F_W [N] : Outport
  wires:
  Drag/1(F_drag [N]) -> Add/2
  Rolling resistance/1(F_Roll [N]) -> Add/1
  Add/1 -> F_W [N]/1
  v [m/s]/1 -> Drag/1(v [m/s])
  Gradient resistance/1(F_slope [N]) -> Add/3
  alpha [rad]/1 -> Gradient resistance/1(alpha [rad]), Rolling resistance/1(alpha [rad])

== system HDVSim_Dual_Fuel_Hybrid_Truck/Active cruise control/Estimate acceleration/Driving resistance without acceleration ==
  v [m/s] : Inport
  alpha [rad] : Inport  Port=2
  Add : Sum  Inputs=+++
  "Drag " : Subsystem
  Gradient resistance : Subsystem
  Rolling resistance : Subsystem
  F_x (resist) [N] : Outport
  wires:
  "Drag "/1(F_drag [N]) -> Add/2
  Rolling resistance/1(F_Roll [N]) -> Add/1
  Add/1 -> F_x (resist) [N]/1  "F_W"
  v [m/s]/1 -> "Drag "/1(v [m/s])
  Gradient resistance/1(F_slope [N]) -> Add/3
  alpha [rad]/1 -> Gradient resistance/1(alpha [rad]), Rolling resistance/1(alpha [rad])

== system HDVSim_Dual_Fuel_Hybrid_Truck/Active cruise control_old/Estimate acceleration/Fahrwiderstaende ohne Beschleunigung ==
  v [m/s] : Inport
  alpha [rad] : Inport  Port=2
  Add : Sum  Inputs=+++
  drag - Luftwiderstand : Subsystem
  grade resistance - Steigungswiderstand : Subsystem
  rolling resistance - Rollwiderstand : Subsystem
  F_x (Widerstand) [N] : Outport
  wires:
  drag - Luftwiderstand/1(F_Luft [N]) -> Add/2
  rolling resistance - Rollwiderstand/1(F_Roll [N]) -> Add/1
  Add/1 -> F_x (Widerstand) [N]/1  "F_W"
  v [m/s]/1 -> drag - Luftwiderstand/1(v [m/s])
  grade resistance - Steigungswiderstand/1(F_Steig [N]) -> Add/3
  alpha [rad]/1 -> grade resistance - Steigungswiderstand/1(alpha [rad]), rolling resistance - Rollwiderstand/1(alpha [rad])

== system HDVSim_Dual_Fuel_Hybrid_Truck/ICE engine/Consumption/Fuel economy [Liter//100km] ==
  abs Diesel consumption [l] : Inport
  Gas consumption [kg] : Inport  Port=2
  s [km] : Inport  Port=3
  Enable : EnablePort
  Divide1 : Product  Inputs=*/
  Divide2 : Product  Inputs=*/
  kg/km->kg/100km : Gain  Gain=100
  l/km->l/100km : Gain  Gain=100
  Diesel consumption l/100km : Outport
  Gas economy [kg/100km] : Outport  Port=2
  wires:
  Divide1/1 -> l/km->l/100km/1
  l/km->l/100km/1 -> Diesel consumption l/100km/1
  abs Diesel consumption [l]/1 -> Divide1/1
  Divide2/1 -> kg/km->kg/100km/1
  kg/km->kg/100km/1 -> Gas economy [kg/100km]/1
  Gas consumption [kg]/1 -> Divide2/1
  s [km]/1 -> Divide2/2, Divide1/2

== system HDVSim_Dual_Fuel_Hybrid_Truck/Transmission/Determine when shifting occurs/Engine torque incoming to the transmission ==
  note: Engine torque
  M_aftr_aux [Nm] : Inport
  n_ICE [rpm] : Inport  Port=2
  "1/min -> 1/s" : Gain  Gain=1/60
  2*pi : Constant  Value=2*pi
  Constant1 : Constant  Value=auxiliary_consumers.power
  M_ICE - M_aux : Sum
  Product1 : Product  Inputs=*//  RndMeth=Zero
  Saturation : Saturate  UpperLimit=inf  LowerLimit=0.001
  M_bfor_aux [Nm] : Outport
  wires:
  M_ICE - M_aux/1 -> M_bfor_aux [Nm]/1
  M_aftr_aux [Nm]/1 -> M_ICE - M_aux/1
  Product1/1 -> M_ICE - M_aux/2
  Constant1/1 -> Product1/1
  2*pi/1 -> Product1/2
  "1/min -> 1/s"/1 -> Product1/3
  n_ICE [rpm]/1 -> Saturation/1
  Saturation/1 -> "1/min -> 1/s"/1

== system HDVSim_Dual_Fuel_Hybrid_Truck/Transmission/Determine when shifting occurs/Gear change recommendation ==
  M_ICE [Nm] : Inport
  n_ICE [rpm] : Inport  Port=2
  alpha : Inport  Port=3
  Constant : Constant  Value=engine.shift_parameter.n1
  Constant1 : Constant  Value=engine.shift_parameter.n3
  Constant2 : Constant  Value=engine.shift_parameter.n2
  Constant3 : Constant  Value=engine.shift_parameter.n6
  Constant4 : Constant  Value=engine.shift_parameter.n5
  Constant5 : Constant  Value=0
  M_max [Nm] : Constant  Value=engine.shift_parameter.M_max
  Switch : Switch  Criteria=u2 > Threshold  Threshold=0.06
  recommend_down_calcbsfc : Subsystem
  recommend_up_calc_bsfc : Subsystem
  recommend_down : Outport
  recommend_up : Outport  Port=2
  wires:
  M_max [Nm]/1 -> recommend_down_calcbsfc/6(M_max [Nm]), recommend_up_calc_bsfc/6(M_max [Nm])  "M_max"
  n_ICE [rpm]/1 -> recommend_down_calcbsfc/1(n), recommend_up_calc_bsfc/5(n)
  M_ICE [Nm]/1 -> recommend_up_calc_bsfc/1(M), recommend_down_calcbsfc/2(M)
  recommend_down_calcbsfc/1(Out1) -> recommend_down/1
  Constant/1 -> recommend_down_calcbsfc/3(n_1)
  Constant1/1 -> recommend_down_calcbsfc/4(n_3)
  Constant2/1 -> recommend_up_calc_bsfc/3(n_2), recommend_down_calcbsfc/5(n_2)
  Constant3/1 -> recommend_up_calc_bsfc/2(n_6)
  Constant4/1 -> recommend_up_calc_bsfc/4(n_5)
  Constant5/1 -> Switch/1
  recommend_up_calc_bsfc/1(recommend_up) -> Switch/3
  Switch/1 -> recommend_up/1
  alpha/1 -> Switch/2

== system HDVSim_Dual_Fuel_Hybrid_Truck/Vehicle/Driving resistances without acceleration/Drag ==
  note: F_Drag = 0.5 * V^2 * rho * A * c_d
  v [m/s] : Inport
  A : Constant  Value=vehicle.frontal_area
  Product2 : Product  Inputs=4  RndMeth=Zero
  c_d : Constant  Value=vehicle.air_drag_coeff
  gain2 : Gain  Gain=0.5
  rho : Constant  Value=ambient.air_density
  v² : Math  Operator=square  SaturateOnIntegerOverflow=on
  F_drag [N] : Outport
  wires:
  v²/1 -> Product2/1
  gain2/1 -> F_drag [N]/1
  v [m/s]/1 -> v²/1
  rho/1 -> Product2/2
  A/1 -> Product2/3
  c_d/1 -> Product2/4
  Product2/1 -> gain2/1

== system HDVSim_Dual_Fuel_Hybrid_Truck/Vehicle/Driving resistances without acceleration/Gradient resistance ==
  note: F_slope = (m_tot * g) * sin(alpha)
  alpha [rad] : Inport
  Add : Sum
  Product7 : Product  RndMeth=Zero
  Trigonometric Function : Trigonometry
  Vehicle mass : Constant  Value=vehicle.mass
  g : Gain  Gain=ambient.gravity
  payload : Constant  Value=vehicle.payload
  F_slope [N] : Outport
  wires:
  alpha [rad]/1 -> Trigonometric Function/1
  Trigonometric Function/1 -> Product7/2
  Product7/1 -> F_slope [N]/1
  g/1 -> Product7/1
  Vehicle mass/1 -> Add/1
  payload/1 -> Add/2
  Add/1 -> g/1

== system HDVSim_Dual_Fuel_Hybrid_Truck/Vehicle/Driving resistances without acceleration/Rolling resistance ==
  note: F_Roll = (m_tot * g) * mu * cos(alpha)
  alpha [rad] : Inport
  Add1 : Sum
  Product7 : Product  Inputs=3  RndMeth=Zero
  Trigonometric Function : Trigonometry  Operator=cos
  g : Gain  Gain=ambient.gravity
  payload : Constant  Value=vehicle.payload
  rolling_resistance_coefficient : Constant  Value=tires.roll_drag_coeff.total
  vehicle mass : Constant  Value=vehicle.mass
  F_Roll [N] : Outport
  wires:
  alpha [rad]/1 -> Trigonometric Function/1
  Product7/1 -> F_Roll [N]/1
  rolling_resistance_coefficient/1 -> Product7/3
  Trigonometric Function/1 -> Product7/1
  g/1 -> Product7/2
  vehicle mass/1 -> Add1/1
  payload/1 -> Add1/2
  Add1/1 -> g/1

== system HDVSim_Dual_Fuel_Hybrid_Truck/Active cruise control/Estimate acceleration/Driving resistance without acceleration/Drag  ==
  note: F_Drag = 0.5 * V^2 * rho * A * c_d
  v [m/s] : Inport
  A : Constant  Value=vehicle.frontal_area
  Product2 : Product  Inputs=4  RndMeth=Zero
  c_d : Constant  Value=vehicle.air_drag_coeff(end)
  gain2 : Gain  Gain=0.5
  rho : Constant  Value=ambient.air_density
  v² : Math  Operator=square  SaturateOnIntegerOverflow=on
  F_drag [N] : Outport
  wires:
  v²/1 -> Product2/1
  gain2/1 -> F_drag [N]/1
  v [m/s]/1 -> v²/1
  rho/1 -> Product2/2
  A/1 -> Product2/3
  Product2/1 -> gain2/1
  c_d/1 -> Product2/4

== system HDVSim_Dual_Fuel_Hybrid_Truck/Active cruise control/Estimate acceleration/Driving resistance without acceleration/Gradient resistance ==
  note: F_slope = (m_tot * g) * sin(alpha)
  alpha [rad] : Inport
  Add : Sum
  Constant1 : Constant  Value=vehicle.payload
  Constant2 : Constant  Value=vehicle.mass
  Product7 : Product  RndMeth=Zero
  Trigonometric Function : Trigonometry
  g : Gain  Gain=ambient.gravity
  F_slope [N] : Outport
  wires:
  alpha [rad]/1 -> Trigonometric Function/1
  Trigonometric Function/1 -> Product7/2
  Product7/1 -> F_slope [N]/1
  g/1 -> Product7/1
  Constant2/1 -> Add/1
  Constant1/1 -> Add/2
  Add/1 -> g/1

== system HDVSim_Dual_Fuel_Hybrid_Truck/Active cruise control/Estimate acceleration/Driving resistance without acceleration/Rolling resistance ==
  note: F_Roll = (m_tot * g) * mu * cos(alpha)
  alpha [rad] : Inport
  Add1 : Sum
  Constant1 : Constant  Value=vehicle.payload
  Constant5 : Constant  Value=tires.roll_drag_coeff.total
  Constant8 : Constant  Value=vehicle.mass
  Product7 : Product  Inputs=3  RndMeth=Zero
  Trigonometric Function : Trigonometry  Operator=cos
  g : Gain  Gain=ambient.gravity
  F_Roll [N] : Outport
  wires:
  alpha [rad]/1 -> Trigonometric Function/1
  Product7/1 -> F_Roll [N]/1
  Constant5/1 -> Product7/3
  Trigonometric Function/1 -> Product7/1
  g/1 -> Product7/2
  Constant8/1 -> Add1/1
  Constant1/1 -> Add1/2
  Add1/1 -> g/1

== system HDVSim_Dual_Fuel_Hybrid_Truck/Active cruise control_old/Estimate acceleration/Fahrwiderstaende ohne Beschleunigung/drag - Luftwiderstand ==
  v [m/s] : Inport
  A : Constant  Value=vehicle.frontal_area
  Product2 : Product  Inputs=4  RndMeth=Zero
  cW : Constant  Value=vehicle.air_drag_coeff
  gain2 : Gain  Gain=0.5
  rho : Constant  Value=ambient.air_density
  v² : Math  Operator=square  SaturateOnIntegerOverflow=on
  F_Luft [N] : Outport
  wires:
  v²/1 -> Product2/1
  gain2/1 -> F_Luft [N]/1
  v [m/s]/1 -> v²/1
  rho/1 -> Product2/2
  A/1 -> Product2/3
  cW/1 -> Product2/4
  Product2/1 -> gain2/1

== system HDVSim_Dual_Fuel_Hybrid_Truck/Active cruise control_old/Estimate acceleration/Fahrwiderstaende ohne Beschleunigung/grade resistance - Steigungswiderstand ==
  alpha [rad] : Inport
  Add : Sum
  Constant1 : Constant  Value=vehicle.payload
  Constant2 : Constant  Value=vehicle.mass
  Product7 : Product  RndMeth=Zero
  Trigonometric Function : Trigonometry
  g : Gain  Gain=ambient.gravity
  F_Steig [N] : Outport
  wires:
  alpha [rad]/1 -> Trigonometric Function/1
  Trigonometric Function/1 -> Product7/2
  Product7/1 -> F_Steig [N]/1
  g/1 -> Product7/1
  Constant2/1 -> Add/1
  Constant1/1 -> Add/2
  Add/1 -> g/1

== system HDVSim_Dual_Fuel_Hybrid_Truck/Active cruise control_old/Estimate acceleration/Fahrwiderstaende ohne Beschleunigung/rolling resistance - Rollwiderstand ==
  alpha [rad] : Inport
  Add1 : Sum
  Constant1 : Constant  Value=vehicle.payload
  Constant5 : Constant  Value=tires.roll_drag_coeff.total
  Constant8 : Constant  Value=vehicle.mass
  Product7 : Product  Inputs=3  RndMeth=Zero
  Trigonometric Function : Trigonometry  Operator=cos
  g : Gain  Gain=ambient.gravity
  F_Roll [N] : Outport
  wires:
  alpha [rad]/1 -> Trigonometric Function/1
  Product7/1 -> F_Roll [N]/1
  Constant5/1 -> Product7/3
  Trigonometric Function/1 -> Product7/1
  g/1 -> Product7/2
  Constant8/1 -> Add1/1
  Constant1/1 -> Add1/2
  Add1/1 -> g/1

== system HDVSim_Dual_Fuel_Hybrid_Truck/Transmission/Determine when shifting occurs/Gear change recommendation/recommend_down_calcbsfc ==
  n : Inport
  M : Inport  Port=2
  n_1 : Inport  Port=3
  n_3 : Inport  Port=4
  n_2 : Inport  Port=5
  M_max [Nm] : Inport  Port=6
  Compare To Zero2 : simulink/Logic and Bit Operations/Compare To Zero  relop=<=  OutDataTypeStr=boolean
  Compare To Zero3 : simulink/Logic and Bit Operations/Compare To Zero  relop=<=  OutDataTypeStr=boolean
  MATLAB Function : MATLAB Function  TreatAsAtomicUnit=on
  Sum1 : Sum  Inputs=+-|
  Sum2 : Sum  Inputs=-+|
  logic2 : Logic  Operator=OR  AllPortsSameDT=off  OutDataTypeStr=boolean
  Out1 : Outport
  wires:
  n_1/1 -> MATLAB Function/3(n_1)  "n_1"
  n_3/1 -> MATLAB Function/4(n_3)
  Sum2/1 -> Compare To Zero2/1
  Sum1/1 -> Compare To Zero3/1
  MATLAB Function/1(g_1) -> Sum2/2
  Compare To Zero3/1 -> logic2/2
  logic2/1 -> Out1/1
  n/1 -> MATLAB Function/1(n), Sum1/1
  n_2/1 -> Sum1/2
  M/1 -> Sum2/1
  M_max [Nm]/1 -> MATLAB Function/2(M_max)
  Compare To Zero2/1 -> logic2/1
